simulink model "lab2"  (R2022a)
settings: Solver=VariableStepAuto  StartTime=0.0  StopTime=1700  RelTol=1e-3
model workspace (MAT data in the model file):
  Mean = 0
  Time = 7.5
  Var = 1
undefined symbols (not defined in the file): m, n
libraries: dspstat3 x1, dspmathops x1
settings Model: ParameterArgumentNames=Time  Creator=Admin  LastModifiedBy=Admin
settings SolverCC: AlgebraicLoopSolver=TrustRegion
settings DataIOCC: SaveOutput=off  SaveTime=off
settings DebuggingCC: UnconnectedInputMsg=warning  UnconnectedOutputMsg=warning  UnconnectedLineMsg=warning  SFMachineParentedDataDiag=warning  ArithmeticOperatorsInVariantConditions=warning
settings SFSimCC: SimUseLocalCustomCode=off  CustomCodeUndefinedFunction=UseInterfaceOnly
settings RTWCC: RTWUseLocalCustomCode=off
settings CodeAppCC: StateflowObjectComments=on

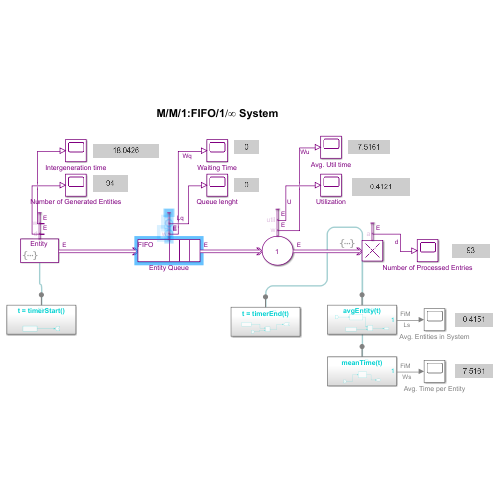
[thumbnail: Simulink's stored preview of the top-level diagram]
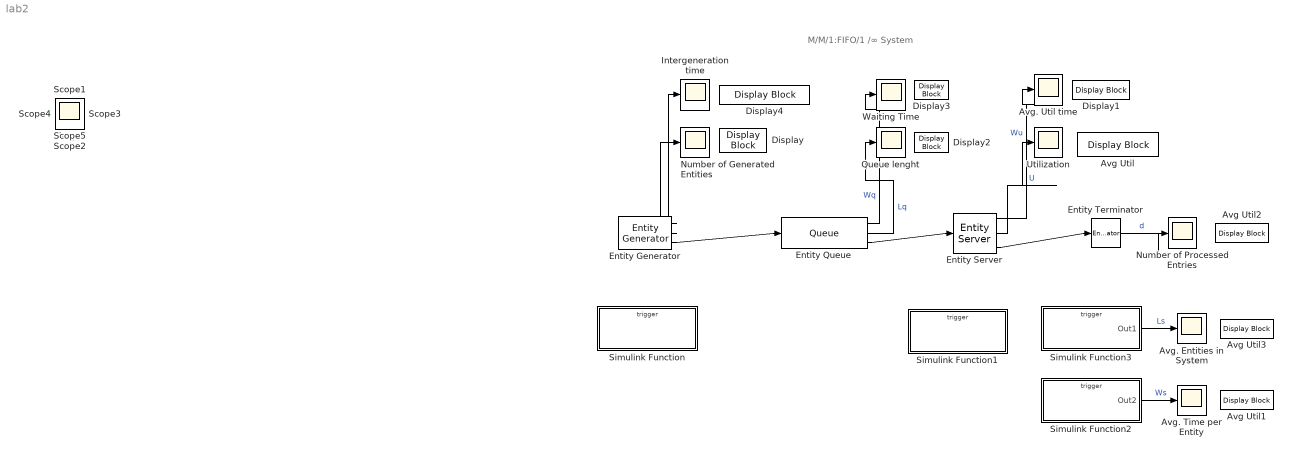
== system lab2 ==
  note: M/M/1:FIFO/1 /∞ System
  Avg Util{,1..3} (4 alike) : DisplayBlock  LabelPosition=Hide  Transparency=1
  Avg. Entities in System : Scope
  Avg. Time per Entity : Scope
  Avg. Util time : Scope
  Display{,1..4} (5 alike) : DisplayBlock  LabelPosition=Hide  Transparency=1
  Entity Generator : EntityGenerator  OutputPortMessageModes=n,n,m  TimeSource=MATLAB action  IntergenerationTimeAction=dt = poissrnd(17.5, 1);  GenerateAction=|  AttributeName=Attribute1|Timer|ServiceTime  AttributeInitialValue=1|1|1  NumberEntitiesDeparted=on  AverageIntergenerationTime=on  EntityType=Structured  EntityTypeName=Entity
      | entity.Timer = timerStart();
      | entity.ServiceTime = exprnd(3);
      settings: OutputPortMap=o0,o2,o3
  Entity Queue : Queue  InputPortMessageModes=m  OutputPortMessageModes=n,n,m  Capacity=1  AverageWait=on  AverageQueueLength=on
      settings: OutputPortMap=o2,o3,o5
  Entity Server : EntityServer  InputPortMessageModes=m  OutputPortMessageModes=n,n,m  Capacity=1  ServiceTimeSource=MATLAB action  ServiceTimeValue=Time  ServiceTimeAction="dt  = poissrnd(7.5, 1);"  AverageWait=on  Utilization=on
      settings: OutputPortMap=o4,o5,o9
  Entity Terminator : EntityTerminator  InputPortMessageModes=m  EntryAction=|  NumberEntitiesArrived=on
      | % Read timer
      | elapsedTime = timerEnd(entity.Timer);
      | 
      | % Compute average
      | meanTime(elapsedTime);
      | avgEntity(elapsedTime);
      settings: OutputPortMap=o0
  Intergeneration time : Scope
  Number of Generated Entities : Scope
  Number of Processed Entries : Scope
  Queue lenght : Scope
  Simulink Function : Subsystem  TreatAsAtomicUnit=on
  Simulink Function1 : Subsystem  TreatAsAtomicUnit=on
  Simulink Function2 : Subsystem  TreatAsAtomicUnit=on
  Simulink Function3 : Subsystem  TreatAsAtomicUnit=on
  Utilization : Scope
  Waiting Time : Scope
  Scope{,1..5} (6 alike) : Scope
  wires:
  Entity Queue/3 -> Entity Server/1
  Entity Server/3 -> Entity Terminator/1
  Entity Queue/1 -> Waiting Time/1  "Wq"
  Entity Queue/2 -> Queue lenght/1  "Lq"
  Entity Server/2 -> Utilization/1  "U"
  Entity Server/1 -> Avg. Util time/1  "Wu"
  Entity Generator/1 -> Number of Generated Entities/1
  Entity Generator/2 -> Intergeneration time/1
  Entity Generator/3 -> Entity Queue/1
  Simulink Function2/1(Out2) -> Avg. Time per Entity/1  "Ws"
  Entity Terminator/1 -> Number of Processed Entries/1  "d"
  Simulink Function3/1(Out1) -> Avg. Entities in System/1  "Ls"

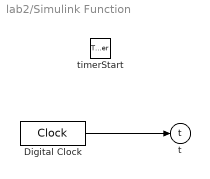
== system lab2/Simulink Function ==
  timerStart : TriggerPort  TriggerType=function-call  IsSimulinkFunction=on  FunctionName=timerStart  FunctionVisibility=scoped  VariantControl=(inherit)
  Digital Clock : DigitalClock  SampleTime=-1
  t : ArgOut  ArgumentName=t
  wires:
  Digital Clock/1 -> t/1

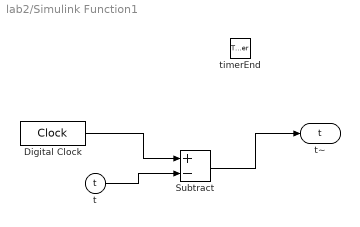
== system lab2/Simulink Function1 ==
  timerEnd : TriggerPort  TriggerType=function-call  IsSimulinkFunction=on  FunctionName=timerEnd  FunctionVisibility=scoped  VariantControl=(inherit)
  Digital Clock : DigitalClock  SampleTime=-1
  Subtract : Sum  Inputs=+-
  t : ArgIn  ArgumentName=t
  t~ : ArgOut  DisableCoverage=on  ArgumentName=t
  wires:
  t/1 -> Subtract/2
  Digital Clock/1 -> Subtract/1
  Subtract/1 -> t~/1

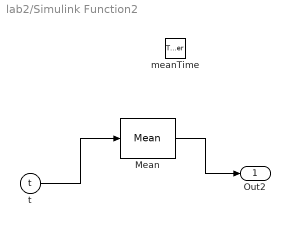
== system lab2/Simulink Function2 ==
  meanTime : TriggerPort  TriggerType=function-call  IsSimulinkFunction=on  FunctionName=meanTime  FunctionVisibility=scoped  VariantControl=(inherit)
  Mean : dspstat3/Mean  run=on  InputProcessing=Columns as channels (frame based)  reset_popup=None  directionMode=Each column  dimension=1  roiEnable=off  roiType=Rectangles  roiPortion=Entire ROI  roiOutput=Individual statistics for each ROI  roiFlag=off  roundingMode=Floor  overflowMode=off  outputDataTypeStr=Inherit: Same as accumulator  outputMin=[]  outputMax=[]  outputLastDataTypeStr=Inherit: Same as accumulator
  t : ArgIn  ArgumentName=t
  Out2 : Outport
  wires:
  t/1 -> Mean/1
  Mean/1 -> Out2/1

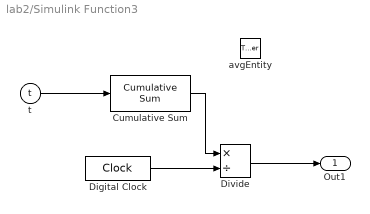
== system lab2/Simulink Function3 ==
  avgEntity : TriggerPort  TriggerType=function-call  IsSimulinkFunction=on  FunctionName=avgEntity  FunctionVisibility=scoped  VariantControl=(inherit)
  Cumulative Sum : dspmathops/Cumulative Sum  dim=Channels (running sum)  InputProcessing=Columns as channels (frame based)  reset_popup=None  roundingMode=Floor  overflowMode=off  outputDataTypeStr=Inherit: Same as accumulator  outputMin=[]  outputMax=[]  outputLastDataTypeStr=Inherit: Same as accumulator
  Digital Clock : DigitalClock  SampleTime=-1
  Divide : Product  Inputs=*/  RndMeth=Zero  SaturateOnIntegerOverflow=on
  t : ArgIn  ArgumentName=t
  Out1 : Outport
  wires:
  Divide/1 -> Out1/1
  Digital Clock/1 -> Divide/2
  t/1 -> Cumulative Sum/1
  Cumulative Sum/1 -> Divide/1
